simulink model "c221007_FCEV_CDCS"  (R2022b)
settings: Solver=ode4  StartTime=1  StopTime=size(Driving_cycle_v_kmph,1)  FixedStep=Auto  RelTol=1e-3  EnableMultiTasking=on
values from neighbouring files (symbols this model uses):
  Bat_eff_chg_average = 0.969    [FCEV_original_data.mat]
  Bat_eff_dis_average = 0.9632    [FCEV_original_data.mat]
  Bat_end_of_life_percent = 20    [FCEV_original_data.mat]
  Bat_I_chg_max = -120    [FCEV_original_data.mat]
  Bat_I_dis_max = 200    [FCEV_original_data.mat]
  Bat_nom_Ic = 2.5    [FCEV_original_data.mat]
  Bat_nom_SOC = 0.35    [FCEV_original_data.mat]
  Bat_nom_temp_oC = 25    [FCEV_original_data.mat]
  Bat_num_pa = 9    [FCEV_original_data.mat]
  Bat_num_se = 97    [FCEV_original_data.mat]
  Bat_ori_C1_chg_F = [397.526659684 455.660832136 435.08783522 460.845064365 457.605812374 417.289828504 416.373906992 359.741413056 321.561704819 1109.14132554 1165.67733205 1135.97600211 ... (72 elements, 9x8)]    [FCEV_original_data.mat]
  Bat_ori_C1_dis_F = [187.121968588 287.083505726 346.448009002 395.529439835 387.517274826 389.973134196 432.856765051 486.92921923 512.158935268 425.990733989 614.68708868 771.472592368 ... (72 elements, 9x8)]    [FCEV_original_data.mat]
  Bat_ori_C2_chg_F = [8748.48589695 7773.35875681 9404.86567646 8934.73981058 8290.58671366 7592.78422269 7759.44623103 7396.59043829 6151.35152293 16187.7227039 11721.8480541 13157.8579836 ... (72 elements, 9x8)]    [FCEV_original_data.mat]
  Bat_ori_C2_dis_F = [2939.81325553 4590.73311898 5504.93546413 5887.5077374 6534.37836712 7765.46899768 10584.7751706 10372.0508438 9238.72693885 5207.86390693 7911.43744944 8879.62137571 ... (72 elements, 9x8)]    [FCEV_original_data.mat]
  Bat_ori_cap_max_Ah = 20.7    [Config_c221218.m]    (also in Config_c230117.m; Config_c230321.m; FCEV_original_data.mat)
  Bat_ori_dUdt4 = [-0.303773584906 -0.249056603774 -0.115094339623 -0.0396226415094 0.0396226415094 0.0641509433962 0.107547169811 0.111320754717 0.0415094339623 0.0547169811321 0.130188679245]    [FCEV_original_data.mat]
  Bat_ori_R0_chg_O = [0.0771669453735 0.0731809311402 0.0726556782939 0.0729965156794 0.0731758310684 0.0742031005051 0.0721266921026 0.0714211058078 0.0714186176143 0.0374124505155 0.0354566732504 0.0345430657188 ... (72 elements, 9x8)]    [FCEV_original_data.mat]
  Bat_ori_R0_dis_O = [0.0819458671157 0.0812429476608 0.0803749674507 0.0805513601722 0.0838629023857 0.0850797840015 0.0829875518672 0.0826388888889 0.0812514106148 0.0428124986417 0.0424658903711 0.0428572670451 ... (72 elements, 9x8)]    [FCEV_original_data.mat]
  Bat_ori_R1_chg_O = [0.114339870884 0.105392753268 0.104421193553 0.109821896183 0.114868279838 0.123333154908 0.129174812826 0.149917249373 0.174896487845 0.0420560161846 0.0390948352938 0.0370122837364 ... (72 elements, 9x8)]    [FCEV_original_data.mat]
  Bat_ori_R1_dis_O = [0.304806399643 0.213604089624 0.171463520004 0.151183840498 0.140630862434 0.128795299077 0.116857791733 0.112567113582 0.106368362501 0.0943235089866 0.0730697254134 0.0611414736086 ... (72 elements, 9x8)]    [FCEV_original_data.mat]
  Bat_ori_R2_chg_O = [0.134518959939 0.17565045702 0.161100627268 0.189032232545 0.205639040497 0.226170473035 0.223651875822 0.181765694192 0.212966950836 0.073628872144 0.0788540822416 0.0792414571734 ... (72 elements, 9x8)]    [FCEV_original_data.mat]
  Bat_ori_R2_dis_O = [0.354968099904 0.285293035102 0.286338708953 0.298763853987 0.248762838155 0.178586175471 0.129047399775 0.188406991173 0.174494800676 0.131839238891 0.123225430215 0.132069033134 ... (72 elements, 9x8)]    [FCEV_original_data.mat]
  Bat_ori_SOC2 = [0 0.001 0.002 0.003 0.004 0.005 0.006 0.007 0.008 0.009 0.01 0.011 ... (1001 elements, 1x1001)]    [FCEV_original_data.mat]
  Bat_ori_SOC4 = [-0.00598301069999 0.0920117618231 0.190864167279 0.289083557951 0.387343788287 0.485011843502 0.5850485992 0.678163031937 0.774810095565 0.876684636119 0.972739524626]    [FCEV_original_data.mat]
  Bat_ori_Uoc_chg_V = [2.4478 2.54923264342 2.6007 2.6383 2.66953057366 2.69636321708 2.7197 2.74042850391 2.75906114733 2.77619379074 2.792 2.80675907757 ... (1001 elements, 1x1001)]    [FCEV_original_data.mat]
  Bat_ori_Uoc_dis_V = [1.9998 2.03916768329 2.24724374236 2.39700902919 2.48767431602 2.5476 2.5882 2.6202 2.64771773167 2.6719 2.6933 2.71251566192 ... (1001 elements, 1x1001)]    [FCEV_original_data.mat]
  Bat_ori_Uoc_V = [2.2238 2.29420016335 2.42397187118 2.5176545146 2.57860244484 2.62198160854 2.65395 2.68031425195 2.7033894395 2.72404689537 2.74265 2.75963736975 ... (1001 elements, 1x1001)]    [FCEV_original_data.mat]
  Bat_single_capacity_nom_Ah = 2.3    [FCEV_original_data.mat]
  Bat_SOC_cs_max = 0.4    [FCEV_original_data.mat]
  Bat_SOC_cs_min = 0.2    [FCEV_original_data.mat]
  Bat_SOC_ini = 0.3    [Config_c22100601.m]    (also in Config_c22100701.m; FCEV_original_data.mat = 0.45)
  Bat_SOC_max = 0.9    [FCEV_original_data.mat]
  Bat_SOC_min = 0.3    [FCEV_original_data.mat]
  Bat_temp_amb_oC = 25    [FCEV_original_data.mat]
  Bat_temp_cool_oC = 25    [FCEV_original_data.mat]
  Bat_U_avg_V = Bat_num_se*mean(Bat_ori_Uoc_V)    [Config_c22100601.m]    (also in Config_c22100701.m)
  DCAC_eff = 0.95    [FCEV_original_data.mat]
  DCDC_ori_eff = [0.95 0.96 0.97 0.976 0.98 0.978 0.973 0.962]    [FCEV_original_data.mat]
  DCDC_ori_power_kW = [0 10 20 30 40 50 60 70]    [FCEV_original_data.mat]
  FC_fuel_mass_ini_kg = 10    [FCEV_original_data.mat]
  FC_ori_eff = [0.1 0.33 0.492 0.533 0.559 0.596 0.591 0.562 0.508]    [FCEV_original_data.mat]
  FC_ori_fuel_rate_gps = [0 0.0505050505051 0.0846883468835 0.117260787992 0.149075730471 0.279642058166 0.423011844332 0.593119810202 0.820209973753]    [FCEV_original_data.mat]
  FC_ori_power_kW = [0 2 5 7.5 10 20 30 40 50]    [FCEV_original_data.mat]
  FC_power_max_kW = 50    [FCEV_original_data.mat]
  FC_power_min_kW = 0    [FCEV_original_data.mat]
  MC_eff_brk_average = 0.810578512397    [FCEV_original_data.mat]
  MC_eff_dri_average = 0.810578512397    [FCEV_original_data.mat]
  MC_inertia = 0.06    [FCEV_original_data.mat]
  MC_ori_eff = [0.7 0.78 0.85 0.86 0.81 0.82 0.79 0.78 0.78 0.78 0.78 0.7 ... (231 elements, 11x21)]    [FCEV_original_data.mat]
  MC_ori_power_brk_req_kW = [0 -28.3912930389 -56.7825860779 -85.1738791168 -113.565172156 -141.956465195 -170.347758234 -198.739051273 -227.130344311 -255.52163735 -283.912930389 0 ... (121 elements, 11x11)]    [FCEV_original_data.mat]
  MC_ori_power_dri_req_kW = [0 0 0 0 0 0 0 0 0 0 0 0 ... (121 elements, 11x11)]    [FCEV_original_data.mat]
  MC_ori_spd_rpm = [0 1000 2000 3000 4000 5000 6000 7000 8000 9000 10000]    [FCEV_original_data.mat]
  MC_ori_trq_brk_max_Nm = [-271.1368 -271.1368 -271.1368 -237.5159 -178.1369 -142.4824 -118.7579 -101.8119 -89.0685 -79.172 -71.1734]    [FCEV_original_data.mat]
  MC_ori_trq_brk_Nm = [-271.136848522 -244.02316367 -216.909478817 -189.795793965 -162.682109113 -135.568424261 -108.454739409 -81.3410545565 -54.2273697044 -27.1136848522 0]    [FCEV_original_data.mat]
  MC_ori_trq_dri_max_Nm = [271.1368 271.1368 271.1368 237.5159 178.1369 142.4824 118.7579 101.8119 89.0685 79.172 71.1734]    [FCEV_original_data.mat]
  MC_ori_trq_dri_Nm = [0 27.1136848522 54.2273697044 81.3410545565 108.454739409 135.568424261 162.682109113 189.795793965 216.909478817 244.02316367 271.136848522]    [FCEV_original_data.mat]
  MC_ori_trq_Nm = [-271.136848522 -244.02316367 -216.909478817 -189.795793965 -162.682109113 -135.568424261 -108.454739409 -81.3410545565 -54.2273697044 -27.1136848522 0 27.1136848522 ... (21 elements, 1x21)]    [FCEV_original_data.mat]
  MC_power_max_kW = 75    [FCEV_original_data.mat]
  MC_spd_max_rpm = 10000    [FCEV_original_data.mat]
  MC_spd_min_rpm = 0    [FCEV_original_data.mat]
  MC_spd_scale = 1    [FCEV_original_data.mat]
  MC_trq_scale = 1    [FCEV_original_data.mat]
  MC_U_min_V = 120    [FCEV_original_data.mat]
  Road_u = 0.75    [FCEV_original_data.mat]
  S_r = floor(max(Sr_SOC_process(:,1))):-1:0    [Config_c22100601.m]    (also in Config_c22100701.m)
  Time_sample = 60    [Driving_cycle_recognition_data.mat]
  Trip_distance_total_km = sum(Driving_cycle_v_kmph(:,2)/3.6)/1000    [Config_c22100601.m]    (also in Config_c22100701.m)
  usd2rmb = 7.116    [Config_c22100601.m]    (also in Config_c22100701.m; Config_c221106.m = 6; Config_c221112.m = 6; Config_c221127.m = 6)
  Veh_air_density_kgpm2 = 1.2    [FCEV_original_data.mat]
  Veh_brk_front = [1 0.6 0.608 0.61 0.618 0.624 0.636 0.645 0.655]    [FCEV_original_data.mat]
  Veh_brk_z = [0.1 0.2 0.3 0.4 0.5 0.6 0.7 0.8 0.9]    [FCEV_original_data.mat]
  Veh_brk_z_max = 0.7    [FCEV_original_data.mat]
  Veh_brk_z_min = 0.1    [FCEV_original_data.mat]
  Veh_coeff_drag = 0.312    [FCEV_original_data.mat]
  Veh_coeff_roll = 0.00863    [FCEV_original_data.mat]
  Veh_final_drive_inertia = 0.1105    [FCEV_original_data.mat]
  Veh_final_drive_ratio = 3.47    [FCEV_original_data.mat]
  Veh_frontal_area_m2 = 2.06    [FCEV_original_data.mat]
  Veh_gravity_acc_ms2 = 9.81    [FCEV_original_data.mat]
  Veh_mass_cargo_kg = 113    [FCEV_original_data.mat]
  Veh_mass_curb_kg = 1157    [FCEV_original_data.mat]
  Veh_mech_eff = 0.9    [FCEV_original_data.mat]
  Veh_rotary_mass_conversion_factor = 1.05    [FCEV_original_data.mat]
  Veh_size_cg_height_m = 0.53    [FCEV_original_data.mat]
  Veh_wheel_inertia = 3.1039    [FCEV_original_data.mat]
  Veh_wheel_radius_m = 0.313    [FCEV_original_data.mat]
  Veh_wt_frac_front = 0.5    [FCEV_original_data.mat]
undefined symbols (not defined in the file or in its folder): alpha, Bat_ori_temp, Sr_e
libraries: neural x10
(part 3 of 5)

== system c221007_FCEV_CDCS/燃料电池模型/FcDegCountingSubSys/Subsystem ==
  Enable : EnablePort
  Add : Sum
  Constant : Constant
  Memory : Memory
  u : Outport
  wires:
  Constant/1 -> Add/1
  Add/1 -> Memory/1
  Memory/1 -> Add/2, u/1

== system c221007_FCEV_CDCS/燃料电池模型/FcDegCountingSubSys/Subsystem1 ==
  Enable : EnablePort
  Add : Sum
  Constant : Constant
  Memory : Memory
  u : Outport
  wires:
  Memory/1 -> u/1, Add/2
  Add/1 -> Memory/1
  Constant/1 -> Add/1

== system c221007_FCEV_CDCS/电池模型/Capacity Degradation Model (Cell)/计算实际寿命 ==
  note: 参考文献：A control-oriented cycle-life model for hybrid electric vehicle lithiumion batteries
  note: Beta
  note: Alpha
  温度 : Inport
  倍率 : Inport  Port=2
  SOC : Inport  Port=3
  -31700+163.3*Ic : Sum  InputSameDT=on  SaturateOnIntegerOverflow=on  OutDataTypeStr=Inherit: Same as first input
  Alpha*SOC+Beta1 : Sum  InputSameDT=on  SaturateOnIntegerOverflow=on  OutDataTypeStr=Inherit: Same as first input
  Alpha3 : Constant  Value=2896.6
  Alpha4 : Constant  Value=2649.5
  Beta3 : Constant  Value=7411.2
  Beta4 : Constant  Value=6022.2
  Constant : Constant  Value=-31500
  Constant1 : Constant  Value=152.5
  Constant2 : Constant  Value=273.15
  Fcn2 : Fcn  Expr=u^(1/0.57)
  Math Function : Math  Operator=reciprocal  SignedPower=on
  Math Function1 : Math  Operator=reciprocal  SignedPower=on
  Math Function2 : Math  SignedPower=on
  R : Constant  Value=8.314
  R*T : Product  InputSameDT=on  RndMeth=Zero  SaturateOnIntegerOverflow=on  OutDataTypeStr=Inherit: Same as first input
  Switch3 : Switch  Criteria=u2 > Threshold  Threshold=0.45
  Switch4 : Switch  Criteria=u2 > Threshold  Threshold=0.45
  severity factor function : Product  InputSameDT=on  RndMeth=Zero  SaturateOnIntegerOverflow=on  OutDataTypeStr=Inherit: Same as first input
  x : Product  InputSameDT=on  RndMeth=Zero  SaturateOnIntegerOverflow=on  OutDataTypeStr=Inherit: Same as first input
  x1 : Product  InputSameDT=on  RndMeth=Zero  SaturateOnIntegerOverflow=on  OutDataTypeStr=Inherit: Same as first input
  x2 : Product  InputSameDT=on  RndMeth=Zero  SaturateOnIntegerOverflow=on  OutDataTypeStr=Inherit: Same as first input
  ×1 : Product  InputSameDT=on  RndMeth=Zero  SaturateOnIntegerOverflow=on  OutDataTypeStr=Inherit: Same as first input
  ℃->开氏温度(绝对温度) : Sum  InputSameDT=on  SaturateOnIntegerOverflow=on  OutDataTypeStr=Inherit: Same as first input
  电池标准状态寿命 : ToWorkspace  VariableName=Bat_life_nom  SampleTime=-1
  电池终止寿命(%) : Constant  Value=Bat_end_of_life_percent
  Bat_life_nom : Outport
  wires:
  R/1 -> R*T/1
  ℃->开氏温度(绝对温度)/1 -> R*T/2
  Constant/1 -> -31700+163.3*Ic/1
  x/1 -> -31700+163.3*Ic/2
  Constant1/1 -> x/1
  -31700+163.3*Ic/1 -> x1/1
  R*T/1 -> Math Function/1
  Math Function/1 -> x1/2
  x1/1 -> Math Function2/1
  温度/1 -> ℃->开氏温度(绝对温度)/1
  Constant2/1 -> ℃->开氏温度(绝对温度)/2
  倍率/1 -> x/2
  Math Function2/1 -> severity factor function/1
  Alpha*SOC+Beta1/1 -> severity factor function/2
  severity factor function/1 -> Math Function1/1
  电池终止寿命(%)/1 -> x2/1
  Math Function1/1 -> x2/2
  x2/1 -> Fcn2/1
  Fcn2/1 -> Bat_life_nom/1, 电池标准状态寿命/1
  SOC/1 -> Switch4/2, ×1/1, Switch3/2
  Alpha4/1 -> Switch3/1
  Alpha3/1 -> Switch3/3
  Beta4/1 -> Switch4/1
  Beta3/1 -> Switch4/3
  Switch3/1 -> ×1/2
  Switch4/1 -> Alpha*SOC+Beta1/2
  ×1/1 -> Alpha*SOC+Beta1/1

== system c221007_FCEV_CDCS/电池模型/Capacity Degradation Model (Cell)/计算电池寿命(标准条件下) ==
  note: 参考文献：A control-oriented cycle-life model for hybrid electric vehicle lithiumion batteries
  note: Beta
  note: Alpha
  标准温度 : Inport
  标准倍率 : Inport  Port=2
  标准SOC : Inport  Port=3
  -31500+152.5*Ic : Sum  InputSameDT=on  SaturateOnIntegerOverflow=on  OutDataTypeStr=Inherit: Same as first input
  Alpha*SOC+Beta : Sum  InputSameDT=on  SaturateOnIntegerOverflow=on  OutDataTypeStr=Inherit: Same as first input
  Alpha3 : Constant  Value=2896.6
  Alpha4 : Constant  Value=2649.5
  Beta3 : Constant  Value=7411.2
  Beta4 : Constant  Value=6022.2
  Constant : Constant  Value=-31500
  Constant1 : Constant  Value=152.5
  Constant2 : Constant  Value=273.15
  Fcn2 : Fcn  Expr=u^(1/0.57)
  Math Function : Math  Operator=reciprocal  SignedPower=on
  Math Function1 : Math  Operator=reciprocal  SignedPower=on
  Math Function2 : Math  SignedPower=on
  R : Constant  Value=8.314
  R*T : Product  InputSameDT=on  RndMeth=Zero  SaturateOnIntegerOverflow=on  OutDataTypeStr=Inherit: Same as first input
  Switch3 : Switch  Criteria=u2 > Threshold  Threshold=0.45
  Switch4 : Switch  Criteria=u2 > Threshold  Threshold=0.45
  severity factor function : Product  InputSameDT=on  RndMeth=Zero  SaturateOnIntegerOverflow=on  OutDataTypeStr=Inherit: Same as first input
  x : Product  InputSameDT=on  RndMeth=Zero  SaturateOnIntegerOverflow=on  OutDataTypeStr=Inherit: Same as first input
  x1 : Product  InputSameDT=on  RndMeth=Zero  SaturateOnIntegerOverflow=on  OutDataTypeStr=Inherit: Same as first input
  x2 : Product  InputSameDT=on  RndMeth=Zero  SaturateOnIntegerOverflow=on  OutDataTypeStr=Inherit: Same as first input
  ×1 : Product  InputSameDT=on  RndMeth=Zero  SaturateOnIntegerOverflow=on  OutDataTypeStr=Inherit: Same as first input
  ℃->开氏温度(绝对温度) : Sum  InputSameDT=on  SaturateOnIntegerOverflow=on  OutDataTypeStr=Inherit: Same as first input
  电池实际状态寿命 : ToWorkspace  VariableName=Bat_life_act  SampleTime=-1
  电池终止寿命(%) : Constant  Value=Bat_end_of_life_percent
  Bat_life_act : Outport
  wires:
  R/1 -> R*T/1
  ℃->开氏温度(绝对温度)/1 -> R*T/2
  Constant/1 -> -31500+152.5*Ic/1
  x/1 -> -31500+152.5*Ic/2
  Constant1/1 -> x/1
  -31500+152.5*Ic/1 -> x1/1
  R*T/1 -> Math Function/1
  Math Function/1 -> x1/2
  x1/1 -> Math Function2/1
  标准温度/1 -> ℃->开氏温度(绝对温度)/1
  Constant2/1 -> ℃->开氏温度(绝对温度)/2
  标准倍率/1 -> x/2
  Math Function2/1 -> severity factor function/1
  Alpha*SOC+Beta/1 -> severity factor function/2
  severity factor function/1 -> Math Function1/1
  电池终止寿命(%)/1 -> x2/1
  Math Function1/1 -> x2/2
  x2/1 -> Fcn2/1
  Fcn2/1 -> Bat_life_act/1, 电池实际状态寿命/1
  标准SOC/1 -> Switch4/2, ×1/1, Switch3/2
  Alpha4/1 -> Switch3/1
  Alpha3/1 -> Switch3/3
  Beta4/1 -> Switch4/1
  Beta3/1 -> Switch4/3
  Switch3/1 -> ×1/2
  Switch4/1 -> Alpha*SOC+Beta/2
  ×1/1 -> Alpha*SOC+Beta/1

== system c221007_FCEV_CDCS/电池模型/Electrical Model/Current calculation ==
  note: #:电池单体水平
  note: R0chg
  note: R0dis
  Voc : Inport
  Rint : Inport  Port=2
  limited output power (W) : Inport  Port=3
  Constant : Constant  Value=Bat_I_chg_max
  Constant1 : Constant  Value=Bat_I_dis_max
  Constant2 : Constant  Value=0
  Demux : Demux  Outputs=2
  Ibty=(Voc-(Voc^2-4RPbty)^.5) ----------------------------- (2*R) : Fcn  Expr=(u[2]-(u[2]^2-4*u[1]*u[3])^.5)/(2*u[3])
  Ibty=(Voc-(Voc^2-4RPbty)^.5) ----------------------------- (2*R)1 : Fcn  Expr=(u[2]-(u[2]^2-4*u[1]*u[3])^.5)/(2*u[3])
  MinMax : MinMax  Inputs=2
  MinMax1 : MinMax  Function=max  Inputs=2
  Mux : Mux  Inputs=2
  Mux1 : Mux  Inputs=3
  Mux2 : Mux  Inputs=3
  Pbat->Pcell : Gain  Gain=1/(Bat_num_pa*Bat_num_se)  SaturateOnIntegerOverflow=on  OutDataTypeStr=Inherit: Same as input  ParamDataTypeStr=Inherit: Same as input
  Scope : Scope
  Scope1 : Scope
  Switch : Switch  Criteria=u2 > Threshold
  Switch1 : Switch  Criteria=u2 > Threshold  SaturateOnIntegerOverflow=off  InputSameDT=off
  Switch2 : Switch  Criteria=u2 > Threshold
  I_dis (A) I_chg (A) Cell : Outport  InitialOutput=0
  I (A) Cell : Outport  Port=2  InitialOutput=0
  wires:
  Rint/1 -> Demux/1
  limited output power (W)/1 -> Pbat->Pcell/1
  Pbat->Pcell/1 -> Switch/1, Switch/2, Switch2/3, Switch2/2, Switch1/2
  Mux1/1 -> Ibty=(Voc-(Voc^2-4RPbty)^.5) ----------------------------- (2*R)/1
  Demux/1 -> Mux1/3
  Voc/1 -> Mux1/2, Mux2/2
  Demux/2 -> Mux2/3
  Mux2/1 -> Ibty=(Voc-(Voc^2-4RPbty)^.5) ----------------------------- (2*R)1/1
  Ibty=(Voc-(Voc^2-4RPbty)^.5) ----------------------------- (2*R)/1 -> MinMax/2
  Constant1/1 -> MinMax/1
  Ibty=(Voc-(Voc^2-4RPbty)^.5) ----------------------------- (2*R)1/1 -> MinMax1/1
  Constant/1 -> MinMax1/2
  MinMax/1 -> Switch1/1, Mux/1
  MinMax1/1 -> Mux/2, Switch1/3
  Mux/1 -> Scope/1, I_dis (A) I_chg (A) Cell/1
  Switch1/1 -> Scope1/1, I (A) Cell/1
  Switch/1 -> Mux1/1
  Switch2/1 -> Mux2/1
  Constant2/1 -> Switch/3, Switch2/1

== system c221007_FCEV_CDCS/电池模型/Electrical Model/Entropic Heat ==
  note: 用于计算可逆热
  T : Inport
  SOC : Inport  Port=2
  Constant : Constant  Value=273
  Ent heat : Product  RndMeth=Zero
  Scope : Scope
  Sum2 : Sum  Inputs=|++
  dudT : Lookup  InputValues=Bat_ori_SOC4  Table=Bat_ori_dUdt4  SaturateOnIntegerOverflow=off
  mV->V : Gain  Gain=1/1000
  HG_ent : Outport
  wires:
  Sum2/1 -> Ent heat/2
  Constant/1 -> Sum2/2
  T/1 -> Sum2/1
  dudT/1 -> Ent heat/1
  Ent heat/1 -> mV->V/1
  SOC/1 -> dudT/1
  mV->V/1 -> Scope/1, HG_ent/1

== system c221007_FCEV_CDCS/电池模型/Electrical Model/Limited power (Battery pack level) ==
  SOC : Inport
  Pbty : Inport  Port=2
  " " : RelationalOperator  Operator=>  OutDataTypeStr=boolean  InputSameDT=off
  " 1" : RelationalOperator  Operator=<  OutDataTypeStr=boolean  InputSameDT=off
  " 3" : Constant  Value=0.95
  Add : Sum
  Constant : Constant  Value=eps
  Constant1 : Constant  Value=eps
  Constant{2..5} (4 alike) : Constant  Value=0
  Logical Operator : Logic  Operator=OR  AllPortsSameDT=off  OutDataTypeStr=boolean
  Logical Operator1 : Logic  AllPortsSameDT=off  OutDataTypeStr=boolean
  Memory1 : Memory  InitialCondition=Bat_SOC_ini  InheritSampleTime=on
  Relational Operator : RelationalOperator  Operator=>  OutDataTypeStr=boolean  InputSameDT=off
  Relational Operator1 : RelationalOperator  OutDataTypeStr=boolean  InputSameDT=off
  Scope : Scope
  Scope1 : Scope  NumInputPorts=2
  Scope2 : Scope  NumInputPorts=2
  Scope3 : Scope
  Switch{,1..3} (4 alike) : Switch  Criteria=u2 > Threshold  Threshold=eps  SaturateOnIntegerOverflow=off  InputSameDT=off
  "Pbty, limited W" : Outport  InitialOutput=0
  wires:
  Memory1/1 -> Relational Operator/1, Relational Operator1/1, Scope3/1
  Constant/1 -> Relational Operator/2
  Relational Operator/1 -> Logical Operator/1
  Switch3/1 -> Scope2/2, " 1"/1, Switch1/3
  Constant1/1 -> " "/2
  " "/1 -> Logical Operator/2
  Logical Operator/1 -> Switch/2
  Constant2/1 -> Switch/3
  " 3"/1 -> Relational Operator1/2
  Relational Operator1/1 -> Logical Operator1/1
  Logical Operator1/1 -> Switch1/2
  Constant3/1 -> Switch1/1
  Constant4/1 -> " 1"/2
  " 1"/1 -> Logical Operator1/2
  Switch2/1 -> Scope2/1, " "/1, Switch/1
  Add/1 -> Scope/1, "Pbty, limited W"/1
  Switch/1 -> Scope1/1, Add/1
  Switch1/1 -> Add/2, Scope1/2
  Pbty/1 -> Switch3/3, Switch3/2, Switch2/1, Switch2/2
  Constant5/1 -> Switch3/1, Switch2/3
  SOC/1 -> Memory1/1

== system c221007_FCEV_CDCS/电池模型/Electrical Model/Max power in W (Battery pack level) ==
  Constant3 : Constant  Value=Bat_I_dis_max
  Constant4 : Constant  Value=Bat_I_chg_max
  Max power in W (Battery pack level)1 : Subsystem
  Mux1 : Mux  Inputs=3
  Mux2 : Mux  Inputs=3
  Product : Product  InputSameDT=on  RndMeth=Zero  SaturateOnIntegerOverflow=on  OutDataTypeStr=Inherit: Same as first input
  Product1 : Product  InputSameDT=on  RndMeth=Zero  SaturateOnIntegerOverflow=on  OutDataTypeStr=Inherit: Same as first input
  R0,cell->R0,bat : Gain  Gain=Bat_num_se/Bat_num_pa  SaturateOnIntegerOverflow=on  OutDataTypeStr=Inherit: Same as input  ParamDataTypeStr=Inherit: Same as input
  R0,cell->R0,bat1 : Gain  Gain=Bat_num_se/Bat_num_pa  SaturateOnIntegerOverflow=on  OutDataTypeStr=Inherit: Same as input  ParamDataTypeStr=Inherit: Same as input
  fun : Fcn  Expr=u[2]-u[1]*u[3]
  fun1 : Fcn  Expr=u[2]-u[1]*u[3]
  max ess discharge pwr : Outport  InitialOutput=0
  max ess charge pwr : Outport  Port=2  InitialOutput=0
  wires:
  [Bat_R0_dis_O] -> R0,cell->R0,bat/1
  [Bat_R0_chg_O] -> R0,cell->R0,bat1/1
  Constant4/1 -> Product1/1, Mux2/1
  Constant3/1 -> Product/1, Mux1/1
  R0,cell->R0,bat/1 -> Mux1/3
  [Bat_Uoc_V] -> Mux2/2, Mux1/2
  Mux1/1 -> fun/1
  R0,cell->R0,bat1/1 -> Mux2/3
  Mux2/1 -> fun1/1
  fun/1 -> Product/2
  Product/1 -> max ess discharge pwr/1
  fun1/1 -> Product1/2
  Product1/1 -> max ess charge pwr/1

== system c221007_FCEV_CDCS/电池模型/Electrical Model/Parameter Lookup2 ==
  note: #Cell层面
  SOC : Inport
  T : Inport  Port=2
  P : Inport  Port=3
  Gain{1..5} (5 alike) : Gain
  Lookup C1 : Subsystem
  Lookup C2 : Subsystem
  Lookup R1 : Subsystem
  Lookup R2 : Subsystem
  Lookup Rs : Subsystem
  Lookup Uoc : Subsystem
  Uoc : Outport
  R1 : Outport  Port=2
  C1 : Outport  Port=3
  R2 : Outport  Port=4
  C2 : Outport  Port=5
  R0 : Outport  Port=6
  wires:
  SOC/1 -> Lookup Rs/1(SOC), Lookup R1/1(SOC), Lookup C1/1(SOC), Lookup Uoc/1(SOC), Lookup C2/1(SOC), Lookup R2/1(SOC1)
  T/1 -> Lookup Rs/2(T), Lookup R1/2(T), Lookup C1/2(T), Lookup C2/2(T), Lookup R2/2(T)
  P/1 -> Lookup R1/3(P), Lookup C1/3(P), Lookup C2/3(P), Lookup Uoc/2(P), Lookup R2/3(P)
  Gain3/1 -> C1/1
  Lookup C2/1(C2) -> Gain4/1
  Gain4/1 -> C2/1
  Gain2/1 -> R2/1
  Lookup R2/1(R2) -> Gain2/1
  Gain1/1 -> R1/1
  Lookup R1/1(R1) -> Gain1/1
  Lookup C1/1(C1) -> Gain3/1
  Lookup Uoc/1(Uoc) -> Gain5/1
  Gain5/1 -> Uoc/1
  Lookup Rs/1(R0) -> R0/1

== system c221007_FCEV_CDCS/电池模型/Electrical Model/SOC Calculation ==
  note: 充电
  note: 放电
  note: #:电池组水平
  I_dis (A) I_chg (A) : Inport
  (sec->hrs) : Gain  Gain=1/3600  SaturateOnIntegerOverflow=on  OutDataTypeStr=Inherit: Same as input  ParamDataTypeStr=Inherit: Same as input
  0 <= SOC <= 1 : Saturate  UpperLimit=1  LowerLimit=eps
  Add5 : Sum  Inputs=-+
  Add6 : Sum  Inputs=-+
  Bat SOC0 : Constant  Value=Bat_SOC_ini
  Bat chg eff : Constant  Value=Bat_eff_chg_average
  Bat dis eff : Constant  Value=Bat_eff_dis_average
  CD/CS mode judgement : Subsystem
  Demux : Demux  Outputs=2
  Divide1 : Product  Inputs=*/
  Divide3 : Product  Inputs=**
  Divide4 : Product  Inputs=*/
  Icell->Ibat : Gain  Gain=Bat_num_pa  SaturateOnIntegerOverflow=on  OutDataTypeStr=Inherit: Same as input  ParamDataTypeStr=Inherit: Same as input
  Icell->Ibat1 : Gain  Gain=Bat_num_pa  SaturateOnIntegerOverflow=on  OutDataTypeStr=Inherit: Same as input  ParamDataTypeStr=Inherit: Same as input
  Integrator1 : Integrator  InitialCondition=eps
  Integrator6 : Integrator
  Integrator7 : Integrator
  Product3 : Product  RndMeth=Zero
  Product4 : Product  RndMeth=Zero
  Q0 : Constant  Value=Bat_ori_cap_max_Ah
  Scope : Scope
  Switch : Switch  Criteria=u2 > Threshold  SaturateOnIntegerOverflow=off  InputSameDT=off
  To Workspace3 : ToWorkspace  VariableName=Energy_bat_consume_kWh  SaveFormat=Timeseries  SampleTime=-1
  Ws->kWh : Gain  Gain=-1/(1000*3600)
  Ws->kWh1 : Gain  Gain=-1/(1000*3600)
  SOC : Outport  InitialOutput=0
  wires:
  0 <= SOC <= 1/1 -> CD/CS mode judgement/1(SOC), SOC/1
  I_dis (A) I_chg (A)/1 -> Scope/1, Demux/1
  Demux/1 -> Icell->Ibat/1
  Demux/2 -> Icell->Ibat1/1
  Divide3/1 -> Switch/2, Product3/1, Switch/1
  Icell->Ibat/1 -> Divide3/1
  Bat dis eff/1 -> Divide3/2
  Bat chg eff/1 -> Divide4/2
  Icell->Ibat1/1 -> Divide4/1
  Divide4/1 -> Product4/2, Switch/3
  Add5/1 -> 0 <= SOC <= 1/1
  [Bat_Uoc_V] -> Product4/1, Product3/2
  Add6/1 -> To Workspace3/1
  Product3/1 -> Integrator6/1
  Integrator6/1 -> Ws->kWh/1
  Ws->kWh/1 -> Add6/1
  Product4/1 -> Integrator7/1
  Integrator7/1 -> Ws->kWh1/1
  Ws->kWh1/1 -> Add6/2
  Switch/1 -> (sec->hrs)/1
  (sec->hrs)/1 -> Integrator1/1
  Integrator1/1 -> Divide1/1
  Q0/1 -> Divide1/2
  Bat SOC0/1 -> Add5/2
  Divide1/1 -> Add5/1

== system c221007_FCEV_CDCS/电池模型/Electrical Model/U0 ==
  R0 : Inport
  I : Inport  Port=2
  Demux : Demux  Outputs=2
  Switch : Switch  Criteria=u2 > Threshold  SaturateOnIntegerOverflow=off  InputSameDT=off
  U0=I*R0 : Product  RndMeth=Zero
  U0 : Outport
  wires:
  I/1 -> U0=I*R0/2, Switch/2
  R0/1 -> Demux/1
  Demux/1 -> Switch/1
  Demux/2 -> Switch/3
  Switch/1 -> U0=I*R0/1
  U0=I*R0/1 -> U0/1

== system c221007_FCEV_CDCS/电池模型/Electrical Model/U1&U1 ==
  note: -V2/(C2*R2)+I/C2
  note: -V1/(C1*R1)+I/C1
  R1 : Inport
  C1 : Inport  Port=2
  R2 : Inport  Port=3
  C2 : Inport  Port=4
  I : Inport  Port=5
  Ib/C1 : Product  Inputs=*/  RndMeth=Zero
  Ib/C2 : Product  Inputs=*/  RndMeth=Zero
  Memory : Memory  InitialCondition=eps  InheritSampleTime=on
  Memory1 : Memory  InitialCondition=eps  InheritSampleTime=on
  R1*C1 : Product  Inputs=**  RndMeth=Zero
  R2*C2 : Product  Inputs=**  RndMeth=Zero
  Scope : Scope  NumInputPorts=2
  Scope1 : Scope
  Sum1 : Sum
  Sum2 : Sum  Inputs=|-+
  Sum3 : Sum  Inputs=+-|
  Sum4 : Sum
  U1/(R1*C1) : Product  Inputs=*/  RndMeth=Zero
  U2/(R2*C2) : Product  Inputs=*/  RndMeth=Zero
  U1 : Outport
  U2 : Outport  Port=2
  wires:
  C1/1 -> R1*C1/1, Ib/C1/2
  I/1 -> Scope1/1, Ib/C2/1, Ib/C1/1
  R1/1 -> R1*C1/2
  R1*C1/1 -> U1/(R1*C1)/2
  U1/(R1*C1)/1 -> Sum3/2
  Ib/C1/1 -> Sum3/1
  R2/1 -> R2*C2/1
  C2/1 -> Ib/C2/2, R2*C2/2
  R2*C2/1 -> U2/(R2*C2)/2
  Ib/C2/1 -> Sum2/2
  U2/(R2*C2)/1 -> Sum2/1
  Memory/1 -> U1/(R1*C1)/1, Sum1/2
  Memory1/1 -> Sum4/1, U2/(R2*C2)/1
  Sum3/1 -> Sum1/1
  Sum1/1 -> Scope/1, Memory/1, U1/1
  Sum2/1 -> Sum4/2
  Sum4/1 -> Scope/2, Memory1/1, U2/1

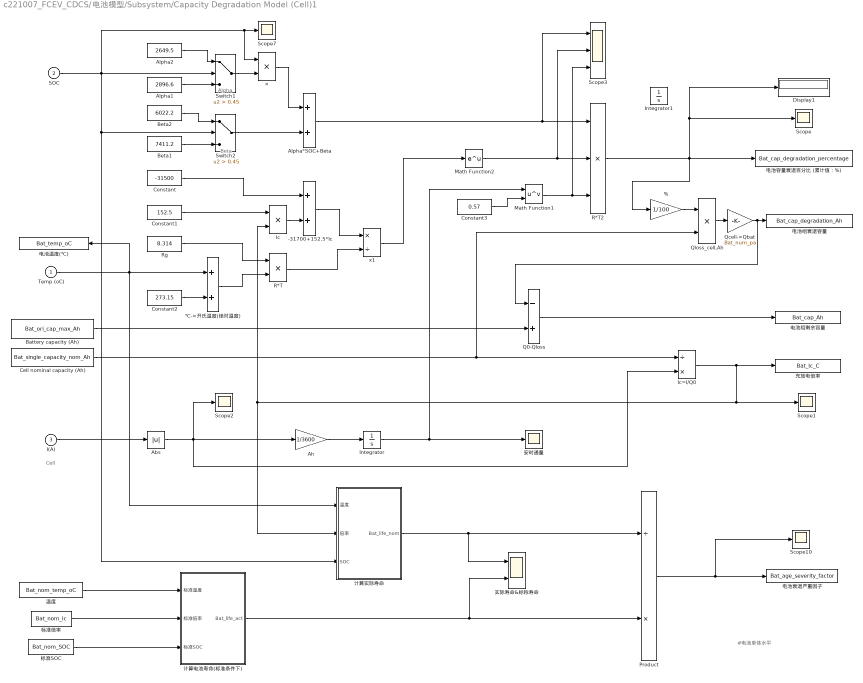
== system c221007_FCEV_CDCS/电池模型/Subsystem/Capacity Degradation Model (Cell)1 ==
  note: Cell
  note: #电池单体水平
  note: Beta
  note: Alpha
  Temp (oC) : Inport
  SOC : Inport  Port=2
  I(A) : Inport  Port=3
  % : Gain  Gain=1/100
  -31700+152.5*Ic : Sum  InputSameDT=on  SaturateOnIntegerOverflow=on  OutDataTypeStr=Inherit: Same as first input
  Abs : Abs  SaturateOnIntegerOverflow=off
  Ah : Gain  Gain=1/3600
  Alpha*SOC+Beta : Sum  InputSameDT=on  SaturateOnIntegerOverflow=on  OutDataTypeStr=Inherit: Same as first input
  Alpha1 : Constant  Value=2896.6
  Alpha2 : Constant  Value=2649.5
  Battery capacity (Ah) : Constant  Value=Bat_ori_cap_max_Ah
  Beta1 : Constant  Value=7411.2
  Beta2 : Constant  Value=6022.2
  Cell nominal capacity (Ah) : Constant  Value=Bat_single_capacity_nom_Ah
  Constant : Constant  Value=-31500
  Constant1 : Constant  Value=152.5
  Constant2 : Constant  Value=273.15
  Constant3 : Constant  Value=0.57
  Display1 : Display
  Ic : Product  InputSameDT=on  RndMeth=Zero  SaturateOnIntegerOverflow=on  OutDataTypeStr=Inherit: Same as first input
  Ic=I/Q0 : Product  Inputs=/*  InputSameDT=on  RndMeth=Zero  SaturateOnIntegerOverflow=on  OutDataTypeStr=Inherit: Same as first input
  Integrator : Integrator  InitialCondition=eps
  Integrator1 : Integrator
  Math Function1 : Math  Operator=pow  SignedPower=on
  Math Function2 : Math  SignedPower=on
  Product : Product  Inputs=/*
  Q0-Qloss : Sum  Inputs=-+  InputSameDT=on  SaturateOnIntegerOverflow=on  OutDataTypeStr=Inherit: Same as first input
  Qcell->Qbat : Gain  Gain=Bat_num_pa  SaturateOnIntegerOverflow=on  OutDataTypeStr=Inherit: Same as input  ParamDataTypeStr=Inherit: Same as input
  Qloss_cell,Ah : Product  InputSameDT=on  RndMeth=Zero  SaturateOnIntegerOverflow=on  OutDataTypeStr=Inherit: Same as first input
  R*T : Product  InputSameDT=on  RndMeth=Zero  SaturateOnIntegerOverflow=on  OutDataTypeStr=Inherit: Same as first input
  R*T2 : Product  Inputs=3  InputSameDT=on  RndMeth=Zero  SaturateOnIntegerOverflow=on  OutDataTypeStr=Inherit: Same as first input
  Rg : Constant  Value=8.314
  Scope{,1..2,7,10} (5 alike) : Scope
  Scope3 : Scope  NumInputPorts=3
  Switch1 : Switch  Criteria=u2 > Threshold  Threshold=0.45
  Switch2 : Switch  Criteria=u2 > Threshold  Threshold=0.45
  x1 : Product  Inputs=*/  InputSameDT=on  RndMeth=Zero  SaturateOnIntegerOverflow=on  OutDataTypeStr=Inherit: Same as first input
  × : Product  InputSameDT=on  RndMeth=Zero  SaturateOnIntegerOverflow=on  OutDataTypeStr=Inherit: Same as first input
  ℃->开氏温度(绝对温度) : Sum  InputSameDT=on  SaturateOnIntegerOverflow=on  OutDataTypeStr=Inherit: Same as first input
  充放电倍率 : ToWorkspace  VariableName=Bat_Ic_C  SampleTime=-1
  安时通量 : Scope
  实际寿命&标称寿命 : Scope  NumInputPorts=2
  标准SOC : Constant  Value=Bat_nom_SOC
  标准倍率 : Constant  Value=Bat_nom_Ic
  温度 : Constant  Value=Bat_nom_temp_oC  VectorParams1D=off
  电池容量衰退百分比 (累计值：%) : ToWorkspace  VariableName=Bat_cap_degradation_percentage  SampleTime=-1
  电池温度(℃) : ToWorkspace  VariableName=Bat_temp_oC  SampleTime=-1
  电池组剩余容量 : ToWorkspace  VariableName=Bat_cap_Ah  SampleTime=-1
  电池组衰退容量 : ToWorkspace  VariableName=Bat_cap_degradation_Ah  SampleTime=-1
  电池衰退严重因子 : ToWorkspace  VariableName=Bat_age_severity_factor  SampleTime=-1
  计算实际寿命 : Subsystem
  计算电池寿命(标准条件下) : Subsystem
  wires:
  SOC/1 -> Switch1/2, Scope7/1, ×/1, Switch2/2, 计算实际寿命/3(SOC)
  Alpha2/1 -> Switch1/1
  Alpha1/1 -> Switch1/3
  Beta2/1 -> Switch2/1
  Beta1/1 -> Switch2/3
  Switch1/1 -> ×/2
  Switch2/1 -> Alpha*SOC+Beta/2
  ×/1 -> Alpha*SOC+Beta/1
  Rg/1 -> R*T/1
  ℃->开氏温度(绝对温度)/1 -> R*T/2
  Ic=I/Q0/1 -> Scope1/1, Ic/2, 计算实际寿命/2(倍率), 充放电倍率/1
  Alpha*SOC+Beta/1 -> R*T2/1, Scope3/1
  Constant/1 -> -31700+152.5*Ic/1
  Ic/1 -> -31700+152.5*Ic/2
  Constant1/1 -> Ic/1
  -31700+152.5*Ic/1 -> x1/1
  R*T/1 -> x1/2
  Math Function2/1 -> R*T2/2, Scope3/2
  x1/1 -> Math Function2/1
  Math Function1/1 -> R*T2/3, Scope3/3
  R*T2/1 -> Scope/1, Display1/1, 电池容量衰退百分比 (累计值：%)/1, %/1
  Abs/1 -> Ic=I/Q0/2, Ah/1, Scope2/1
  Integrator/1 -> Math Function1/1, 安时通量/1
  Temp (oC)/1 -> 计算实际寿命/1(温度), 电池温度(℃)/1, ℃->开氏温度(绝对温度)/1
  Constant2/1 -> ℃->开氏温度(绝对温度)/2
  %/1 -> Qloss_cell,Ah/1
  温度/1 -> 计算电池寿命(标准条件下)/1(标准温度)
  标准倍率/1 -> 计算电池寿命(标准条件下)/2(标准倍率)
  标准SOC/1 -> 计算电池寿命(标准条件下)/3(标准SOC)
  Product/1 -> 电池衰退严重因子/1, Scope10/1
  计算实际寿命/1(Bat_life_nom) -> 实际寿命&标称寿命/1, Product/1
  计算电池寿命(标准条件下)/1(Bat_life_act) -> Product/2, 实际寿命&标称寿命/2
  I(A)/1 -> Abs/1
  Cell nominal capacity (Ah)/1 -> Qloss_cell,Ah/2, Ic=I/Q0/1
  Qcell->Qbat/1 -> Q0-Qloss/1, 电池组衰退容量/1
  Qloss_cell,Ah/1 -> Qcell->Qbat/1
  Battery capacity (Ah)/1 -> Q0-Qloss/2
  Q0-Qloss/1 -> 电池组剩余容量/1
  Ah/1 -> Integrator/1
  Constant3/1 -> Math Function1/2

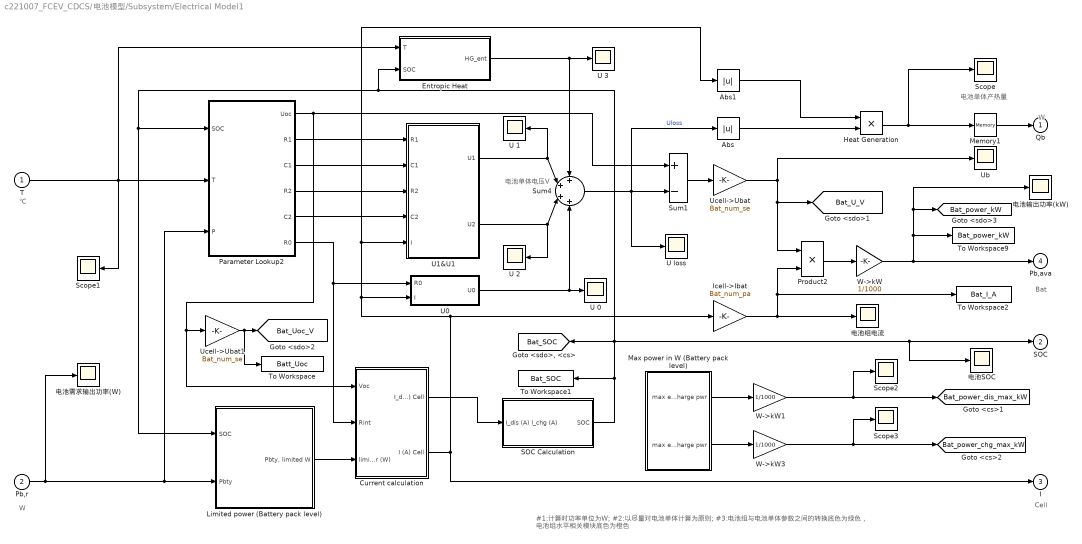
== system c221007_FCEV_CDCS/电池模型/Subsystem/Electrical Model1 ==
  note: Bat
  note: Cell
  note: W
  note: ℃
  note: #1:计算时功率单位为W;
      | #2:以尽量对电池单体计算为原则;
      | #3:电池组与电池单体参数之间的转换底色为绿色， 电池组水平相关模块底色为橙色
  note: W
  note: 电池单体产热量
  note: 电池单体电压V
  T : Inport
  Pb,r : Inport  Port=2
  Abs : Abs  SaturateOnIntegerOverflow=off
  Abs1 : Abs  SaturateOnIntegerOverflow=off
  Current calculation : Subsystem
  Entropic Heat : Subsystem
  Heat Generation : Product  RndMeth=Zero
  Icell->Ibat : Gain  Gain=Bat_num_pa  SaturateOnIntegerOverflow=on  OutDataTypeStr=Inherit: Same as input  ParamDataTypeStr=Inherit: Same as input
  Limited power (Battery pack level) : Subsystem
  Max power in W (Battery pack level) : Subsystem
  Memory1 : Memory  InheritSampleTime=on
  Parameter Lookup2 : Subsystem
  Product2 : Product  RndMeth=Zero
  SOC Calculation : Subsystem
  Scope{,1..3} (4 alike) : Scope
  Sum1 : Sum  Inputs=+-
  Sum4 : Sum  Inputs=++++
  To Workspace : ToWorkspace  VariableName=Batt_Uoc  SaveFormat=Timeseries  SampleTime=-1
  To Workspace1 : ToWorkspace  VariableName=Bat_SOC  SampleTime=-1
  To Workspace2 : ToWorkspace  VariableName=Bat_I_A  SampleTime=-1
  To Workspace9 : ToWorkspace  VariableName=Bat_power_kW  SampleTime=-1
  U {0..3} (4 alike) : Scope
  U loss : Scope
  U0 : Subsystem
  U1&U1 : Subsystem
  Ub : Scope
  Ucell->Ubat : Gain  Gain=Bat_num_se  SaturateOnIntegerOverflow=on  OutDataTypeStr=Inherit: Same as input  ParamDataTypeStr=Inherit: Same as input
  Ucell->Ubat1 : Gain  Gain=Bat_num_se  SaturateOnIntegerOverflow=on  OutDataTypeStr=Inherit: Same as input  ParamDataTypeStr=Inherit: Same as input
  W->kW : Gain  Gain=1/1000  SaturateOnIntegerOverflow=on  OutDataTypeStr=Inherit: Same as input  ParamDataTypeStr=Inherit: Same as input
  W->kW1 : Gain  Gain=1/1000  SaturateOnIntegerOverflow=on  OutDataTypeStr=Inherit: Same as input  ParamDataTypeStr=Inherit: Same as input
  W->kW3 : Gain  Gain=1/1000  SaturateOnIntegerOverflow=on  OutDataTypeStr=Inherit: Same as input  ParamDataTypeStr=Inherit: Same as input
  电池SOC : Scope
  电池组电流 : Scope
  电池输出功率(kW) : Scope
  电池需求输出功率(W) : Scope
  Qb : Outport  InitialOutput=0
  SOC : Outport  Port=2  InitialOutput=0
  I : Outport  Port=3  InitialOutput=0
  Pb,ava : Outport  Port=4  InitialOutput=0
  tag scope: Bat_SOC=global, Bat_U_V=global, Bat_Uoc_V=global, Bat_power_chg_max_kW=global, Bat_power_dis_max_kW=global, Bat_power_kW=global
  wires:
  Parameter Lookup2/2(R1) -> U1&U1/1(R1)
  Parameter Lookup2/3(C1) -> U1&U1/2(C1)
  Parameter Lookup2/4(R2) -> U1&U1/3(R2)
  Parameter Lookup2/5(C2) -> U1&U1/4(C2)
  Parameter Lookup2/6(R0) -> U0/1(R0), Current calculation/2(Rint)
  U1&U1/1(U1) -> Sum4/2, U 1/1
  U1&U1/2(U2) -> U 2/1, Sum4/3
  Ucell->Ubat/1 -> Product2/1, [Bat_U_V], Ub/1
  Entropic Heat/1(HG_ent) -> U 3/1, Sum4/1
  Product2/1 -> W->kW/1
  W->kW/1 -> 电池输出功率(kW)/1, [Bat_power_kW], To Workspace9/1, Pb,ava/1
  Memory1/1 -> Qb/1
  Heat Generation/1 -> Scope/1, Memory1/1
  Current calculation/1(I_dis (A) I_chg (A) Cell) -> SOC Calculation/1(I_dis (A) I_chg (A))
  T/1 -> Scope1/1, Entropic Heat/1(T), Parameter Lookup2/2(T)
  Pb,r/1 -> 电池需求输出功率(W)/1, Limited power (Battery pack level)/2(Pbty), Parameter Lookup2/3(P)
  Icell->Ibat/1 -> Product2/2, To Workspace2/1, 电池组电流/1
  W->kW1/1 -> Scope2/1, [Bat_power_dis_max_kW]
  W->kW3/1 -> Scope3/1, [Bat_power_chg_max_kW]
  Max power in W (Battery pack level)/1(max ess discharge pwr) -> W->kW1/1
  Max power in W (Battery pack level)/2(max ess charge pwr) -> W->kW3/1
  Parameter Lookup2/1(Uoc) -> Sum1/1, Ucell->Ubat1/1, Current calculation/1(Voc)
  Ucell->Ubat1/1 -> To Workspace/1, [Bat_Uoc_V]
  Limited power (Battery pack level)/1("Pbty, limited W") -> Current calculation/3(limited output power (W))
  SOC Calculation/1(SOC) -> 电池SOC/1, SOC/1, [Bat_SOC], Entropic Heat/2(SOC), Limited power (Battery pack level)/1(SOC), Parameter Lookup2/1(SOC), To Workspace1/1
  Current calculation/2(I (A) Cell) -> Abs1/1, U1&U1/5(I), U0/2(I), Icell->Ibat/1, I/1
  U0/1(U0) -> U 0/1, Sum4/4
  Sum4/1 -> U loss/1, Abs/1, Sum1/2  "Uloss"
  Sum1/1 -> Ucell->Ubat/1
  Abs/1 -> Heat Generation/2
  Abs1/1 -> Heat Generation/1

== system c221007_FCEV_CDCS/电池模型/Subsystem/Thermal Model1 ==
  note: 需要设置温度初始值
  note: W
  note: Tf
  note: (k)
  note: 冷却液温度 ℃
  note: ℃
  note: ℃
  Qb : Inport
  (1-1/RsCs-1/RcCs)*Ts(k-1) : Product  Inputs=**  RndMeth=Zero
  (RC*Cc-1)*Tc(k-1)/RcCc : Product  Inputs=**  RndMeth=Zero
  (RC*Cc-1)/RcCc : Product  Inputs=*/  RndMeth=Zero
  Calculation : Subsystem
  Constant : Constant  Value=273
  Constant3 : Constant
  Math Function : Math  Operator=reciprocal  SignedPower=on
  Math Function1 : Math  Operator=reciprocal  SignedPower=on
  Qb(k-1)/Cc : Product  Inputs=*/  RndMeth=Zero
  Sum10 : Sum  Inputs=+++
  Sum11 : Sum  Inputs=+--|
  Sum3 : Sum  Inputs=+++
  Sum4 : Sum  Inputs=+-|
  Sum5 : Sum  Inputs=|+-
  Sum7 : Sum  Inputs=++|
  Sum9 : Sum  Inputs=-+|
  Tc (K) : Scope
  Tc (℃) : Scope
  Tc(k-1) : Memory  InitialCondition=Bat_temp_amb_oC+273.15  InheritSampleTime=on
  Tc(k-1)/RcCs : Product  Inputs=*/  RndMeth=Zero
  Tf/RsCs : Product  Inputs=*/  RndMeth=Zero
  Tf1 : Constant  Value=Bat_temp_cool_oC
  Ts (K) : Scope
  Ts (℃) : Scope
  Ts(k-1) : Memory  InitialCondition=Bat_temp_amb_oC+273.15  InheritSampleTime=on
  Ts(k-1)/RcCc : Product  Inputs=*/  RndMeth=Zero
  Tc. : Outport
  Ts. : Outport  Port=2
  wires:
  Calculation/1(Cc) -> Qb(k-1)/Cc/2
  Calculation/2(RcCc) -> (RC*Cc-1)/RcCc/2, Ts(k-1)/RcCc/2, Sum4/1
  Constant3/1 -> Sum11/1, Sum4/2
  Sum4/1 -> (RC*Cc-1)/RcCc/1
  Qb(k-1)/Cc/1 -> Sum3/1
  Ts(k-1)/RcCc/1 -> Sum3/2
  Tf1/1 -> Sum7/2
  Calculation/3(RsCs) -> Tf/RsCs/2, Math Function/1
  Sum7/1 -> Tf/RsCs/1
  Tf/RsCs/1 -> Sum10/1
  Calculation/4(RcCs) -> Tc(k-1)/RcCs/2, Math Function1/1
  Math Function1/1 -> Sum11/2
  Math Function/1 -> Sum11/3
  (1-1/RsCs-1/RcCs)*Ts(k-1)/1 -> Sum10/2
  Sum11/1 -> (1-1/RsCs-1/RcCs)*Ts(k-1)/1
  Tc(k-1)/RcCs/1 -> Sum10/3
  Sum3/1 -> Sum5/1, Tc(k-1)/1, Tc (K)/1
  Constant/1 -> Sum9/1, Sum5/2, Sum7/1
  Sum5/1 -> Tc (℃)/1, Tc./1
  Sum10/1 -> Sum9/2, Ts(k-1)/1, Ts (K)/1
  Sum9/1 -> Ts./1, Ts (℃)/1
  Ts(k-1)/1 -> Ts(k-1)/RcCc/1, (1-1/RsCs-1/RcCs)*Ts(k-1)/2
  (RC*Cc-1)*Tc(k-1)/RcCc/1 -> Sum3/3
  (RC*Cc-1)/RcCc/1 -> (RC*Cc-1)*Tc(k-1)/RcCc/1
  Tc(k-1)/1 -> Tc(k-1)/RcCs/1, (RC*Cc-1)*Tc(k-1)/RcCc/2
  Qb/1 -> Qb(k-1)/Cc/1

== system c221007_FCEV_CDCS/电池模型/Thermal Model/Calculation ==
  Cc1 : Constant  Value=62.7
  Cs : Constant  Value=4.5
  "Rc " : Constant  Value=1.94
  Rc*Cc : Product  Inputs=**  RndMeth=Zero
  Rc*Cs : Product  Inputs=**  RndMeth=Zero
  Rs : Constant  Value=3.19
  Rs*Cs : Product  Inputs=**  RndMeth=Zero
  Cc : Outport
  RcCc : Outport  Port=2
  RsCs : Outport  Port=3
  RcCs : Outport  Port=4
  wires:
  Cc1/1 -> Cc/1, Rc*Cc/1
  "Rc "/1 -> Rc*Cc/2, Rc*Cs/1
  Rc*Cc/1 -> RcCc/1
  Cs/1 -> Rs*Cs/1, Rc*Cs/2
  Rs/1 -> Rs*Cs/2
  Rc*Cs/1 -> RcCs/1
  Rs*Cs/1 -> RsCs/1

== system c221007_FCEV_CDCS/能量管理策略 (ECMS+SQP)/Collection/    DC_type ==
  In1 : Inport
  Enable : EnablePort
  Out1 : Outport
  wires:
  In1/1 -> Out1/1

== system c221007_FCEV_CDCS/能量管理策略 (ECMS+SQP)/Collection/Bat_SOC ==
  In1 : Inport
  Enable : EnablePort
  Out1 : Outport
  wires:
  In1/1 -> Out1/1

== system c221007_FCEV_CDCS/能量管理策略 (ECMS+SQP)/Collection/Bat_SOC_max ==
  In1 : Inport
  Enable : EnablePort
  Out1 : Outport
  wires:
  In1/1 -> Out1/1

== system c221007_FCEV_CDCS/能量管理策略 (ECMS+SQP)/Collection/Bat_SOC_min ==
  In1 : Inport
  Enable : EnablePort
  Out1 : Outport
  wires:
  In1/1 -> Out1/1

== system c221007_FCEV_CDCS/能量管理策略 (ECMS+SQP)/Collection/Bat_SOC_ref ==
  In1 : Inport
  Enable : EnablePort
  Out1 : Outport
  wires:
  In1/1 -> Out1/1

== system c221007_FCEV_CDCS/能量管理策略 (ECMS+SQP)/Collection/Bat_U_avg_V ==
  In1 : Inport
  Enable : EnablePort
  Out1 : Outport
  wires:
  In1/1 -> Out1/1

== system c221007_FCEV_CDCS/能量管理策略 (ECMS+SQP)/Collection/Bat_cap_Ah ==
  In1 : Inport
  Enable : EnablePort
  Out1 : Outport
  wires:
  In1/1 -> Out1/1

== system c221007_FCEV_CDCS/能量管理策略 (ECMS+SQP)/Collection/Bat_power_max_kW ==
  In1 : Inport
  Enable : EnablePort
  Out1 : Outport
  wires:
  In1/1 -> Out1/1

== system c221007_FCEV_CDCS/能量管理策略 (ECMS+SQP)/Collection/Bat_power_min_kW ==
  In1 : Inport
  Enable : EnablePort
  Out1 : Outport
  wires:
  In1/1 -> Out1/1

== system c221007_FCEV_CDCS/能量管理策略 (ECMS+SQP)/Collection/DCAC_eff ==
  In1 : Inport
  Enable : EnablePort
  Out1 : Outport
  wires:
  In1/1 -> Out1/1

== system c221007_FCEV_CDCS/能量管理策略 (ECMS+SQP)/Collection/FC_power_max_kW ==
  In1 : Inport
  Enable : EnablePort
  Out1 : Outport
  wires:
  In1/1 -> Out1/1

== system c221007_FCEV_CDCS/能量管理策略 (ECMS+SQP)/Collection/FC_power_min_kW ==
  In1 : Inport
  Enable : EnablePort
  Out1 : Outport
  wires:
  In1/1 -> Out1/1

== system c221007_FCEV_CDCS/能量管理策略 (ECMS+SQP)/Collection/MC_power_req_kW ==
  In1 : Inport
  Enable : EnablePort
  Out1 : Outport
  wires:
  In1/1 -> Out1/1

== system c221007_FCEV_CDCS/能量管理策略 (ECMS+SQP)/Collection/X_r_km ==
  In1 : Inport
  Enable : EnablePort
  Out1 : Outport
  wires:
  In1/1 -> Out1/1

== system c221007_FCEV_CDCS/能量管理策略 (ECMS+SQP)/Collection/alpha ==
  In1 : Inport
  Enable : EnablePort
  Out1 : Outport
  wires:
  In1/1 -> Out1/1

== system c221007_FCEV_CDCS/能量管理策略 (ECMS+SQP)/FC on/Subsystem ==
  in_1 : Inport
  Constant1 : Constant  Value=n
  Integrator : Integrator
  Product : Product  Inputs=*/  InputSameDT=on  RndMeth=Zero  SaturateOnIntegerOverflow=on  OutDataTypeStr=Inherit: Same as first input
  Sum : Sum  Inputs=+-  InputSameDT=on  SaturateOnIntegerOverflow=on  OutDataTypeStr=Inherit: Same as first input
  Transport Delay : TransportDelay  DelayTime=n
  out_1 : Outport  InitialOutput=0
  wires:
  Integrator/1 -> Sum/1, Transport Delay/1
  Transport Delay/1 -> Sum/2
  Sum/1 -> Product/1
  in_1/1 -> Integrator/1
  Product/1 -> out_1/1
  Constant1/1 -> Product/2

== system c221007_FCEV_CDCS/能量管理策略 (ECMS+SQP)/FC on/dt ==
  Clock : Clock
  Memory1 : Memory  InitialCondition=-1
  Sum1 : Sum  Inputs=+-  InputSameDT=on  SaturateOnIntegerOverflow=on  OutDataTypeStr=Inherit: Same as first input
  out_1 : Outport  InitialOutput=0
  wires:
  Clock/1 -> Sum1/1, Memory1/1
  Memory1/1 -> Sum1/2
  Sum1/1 -> out_1/1

== system c221007_FCEV_CDCS/能量管理策略 (ECMS+SQP)/FC on/just shut down ==
  state : Inport
  Logical Operator : Logic
  Logical Operator1 : Logic  Operator=NOT  Inputs=1
  Memory1 : Memory  InitialCondition=1  InheritSampleTime=on
  trigger : Outport  InitialOutput=0
  wires:
  Logical Operator1/1 -> Logical Operator/1
  state/1 -> Logical Operator1/1, Memory1/1
  Memory1/1 -> Logical Operator/2
  Logical Operator/1 -> trigger/1

== system c221007_FCEV_CDCS/能量管理策略 (ECMS+SQP)/FC on/no-lag Reset Integrator ==
  in_1 : Inport
  in_2 : Inport  Port=2
  in_3 : Inport  Port=3
  Constant : Constant  Value=0
  Memory : Memory  InitialCondition=initval
  Product : Product  InputSameDT=on  RndMeth=Zero  SaturateOnIntegerOverflow=on  OutDataTypeStr=Inherit: Same as first input
  Sum : Sum  InputSameDT=on  SaturateOnIntegerOverflow=on  OutDataTypeStr=Inherit: Same as first input
  Switch : Switch  Threshold=eps
  dt : Subsystem
  in_2==0 : RelationalOperator  Operator===
  out_1 : Outport  InitialOutput=0
  wires:
  in_3/1 -> Switch/3
  in_2/1 -> in_2==0/1
  in_1/1 -> Product/2
  dt/1(out_1) -> Product/1
  Product/1 -> Sum/2
  Memory/1 -> Sum/1
  Sum/1 -> Switch/1
  Switch/1 -> out_1/1, Memory/1
  in_2==0/1 -> Switch/2
  Constant/1 -> in_2==0/2

== system c221007_FCEV_CDCS/能量管理策略 (ECMS+SQP)/SQP/Power limitation ==
  Add1 : Sum  Inputs=+-
  Add2 : Sum  Inputs=-+
  MinMax : MinMax  Function=max  Inputs=2
  Pfc_min : Constant  Value=FC_power_max_kW
  Relational Operator4 : RelationalOperator  OutDataTypeStr=boolean  InputSameDT=off
  SOC_min1 : Constant  Value=Bat_SOC_min
  Saturation1 : Saturate  UpperLimit=FC_power_max_kW  LowerLimit=FC_power_min_kW  LinearizeAsGain=off
  Switch2 : Switch  Threshold=0.1  SaturateOnIntegerOverflow=off  InputSameDT=off
  Switch3 : Switch  Threshold=0.1  SaturateOnIntegerOverflow=off  InputSameDT=off
  wires:
  Relational Operator4/1 -> Switch3/2, Switch2/2
  SOC_min1/1 -> Relational Operator4/2
  ? -> Switch2/1
  ? -> Switch3/1, Add2/2, Add1/1
  Pfc_min/1 -> Add1/2
  MinMax/1 -> Add2/1, Switch2/3
  Add1/1 -> MinMax/2
  Saturation1/1 -> Switch3/3
  Add2/1 -> Saturation1/1
  [Bat_SOC] -> Relational Operator4/1
  [Bat_power_chg_max_kW] -> MinMax/1

== system c221007_FCEV_CDCS/行驶工况相关/Custom Neural Network/Layer 1 ==
  "p{1}" : Inport  PortDimensions=3
      mask Display: e = 0.06;c1 = [120 230 180]/255;c2 = ([120 230 180]+0)/(256+128);c3 = ([120 230 180]+128)/(256+128);patch([0 1 1 0],[0 0 1 1],c1);patch([0 1 1 1-e 1-e 0+e],[0 0 1 1-e 0+e 0+e],c2);patch([0 0 1 1-e 0+e 0+e],[0 1 1 1-e 1-e 0+e],c3);plot([0 1 1 0 0],[0 0 1 1 0]);
  Delays 1 : Subsystem
      mask Display: e = 0.06;c1 = [120 150 230]/255;c2 = ([120 150 230]+0)/383;c3 = ([120 150 230]+128)/383;patch([0 1 1 0],[0 0 1 1],c1);patch([0 1 1 1-e 1-e 0+e],[0 0 1 1-e 0+e 0+e],c2);patch([0 0 1 1-e 0+e 0+e],[0 1 1 1-e 1-e 0+e],c3);plot([0 1 1 0 0],[0 0 1 1 0]);disp('0');
  "IW{1,1}" : Subsystem
      mask Display: e = 0.06;c1 = [120 150 230]/255;c2 = ([120 150 230]+0)/383;c3 = ([120 150 230]+128)/383;patch([0 1 1 0],[0 0 1 1],c1);patch([0 1 1 1-e 1-e 0+e],[0 0 1 1-e 0+e 0+e],c2);patch([0 0 1 1-e 0+e 0+e],[0 1 1 1-e 1-e 0+e],c3);plot([0 1 1 0 0],[0 0 1 1 0]);disp('W');
  compet : neural/Transfer Functions/compet  layer_size=5
  netsum : Gain  SaturateOnIntegerOverflow=on  OutDataTypeStr=Inherit: Same as input  ParamDataTypeStr=Inherit: Same as input
      mask Display: e = 0.06;c1 = [120 150 230]/255;c2 = ([120 150 230]+0)/383;c3 = ([120 150 230]+128)/383;patch([0 1 1 0],[0 0 1 1],c1);patch([0 1 1 1-e 1-e 0+e],[0 0 1 1-e 0+e 0+e],c2);patch([0 0 1 1-e 0+e 0+e],[0 1 1 1-e 1-e 0+e],c3);plot([0 1 1 0 0],[0 0 1 1 0]);disp('+');
  "a{1}" : Outport  InitialOutput=[0;0;0;0;0]
      mask Display: e = 0.06;c1 = [120 230 180]/255;c2 = ([120 230 180]+0)/(256+128);c3 = ([120 230 180]+128)/(256+128);patch([0 1 1 0],[0 0 1 1],c1);patch([0 1 1 1-e 1-e 0+e],[0 0 1 1-e 0+e 0+e],c2);patch([0 0 1 1-e 0+e 0+e],[0 1 1 1-e 1-e 0+e],c3);plot([0 1 1 0 0],[0 0 1 1 0]);
  wires:
  "p{1}"/1 -> Delays 1/1("p{1}")
  Delays 1/1("pd{1,1}") -> "IW{1,1}"/1("pd{1,1}")
  "IW{1,1}"/1("iz{1,1}") -> netsum/1
  netsum/1 -> compet/1
  compet/1 -> "a{1}"/1

== system c221007_FCEV_CDCS/行驶工况相关/Custom Neural Network/Layer 2 ==
  "a{1} " : Inport  PortDimensions=5
      mask Display: e = 0.06;c1 = [120 230 180]/255;c2 = ([120 230 180]+0)/(256+128);c3 = ([120 230 180]+128)/(256+128);patch([0 1 1 0],[0 0 1 1],c1);patch([0 1 1 1-e 1-e 0+e],[0 0 1 1-e 0+e 0+e],c2);patch([0 0 1 1-e 0+e 0+e],[0 1 1 1-e 1-e 0+e],c3);plot([0 1 1 0 0],[0 0 1 1 0]);
  Delays 1 : Subsystem
      mask Display: e = 0.06;c1 = [120 150 230]/255;c2 = ([120 150 230]+0)/383;c3 = ([120 150 230]+128)/383;patch([0 1 1 0],[0 0 1 1],c1);patch([0 1 1 1-e 1-e 0+e],[0 0 1 1-e 0+e 0+e],c2);patch([0 0 1 1-e 0+e 0+e],[0 1 1 1-e 1-e 0+e],c3);plot([0 1 1 0 0],[0 0 1 1 0]);disp('0');
  "LW{2,1}" : Subsystem
      mask Display: e = 0.06;c1 = [120 150 230]/255;c2 = ([120 150 230]+0)/383;c3 = ([120 150 230]+128)/383;patch([0 1 1 0],[0 0 1 1],c1);patch([0 1 1 1-e 1-e 0+e],[0 0 1 1-e 0+e 0+e],c2);patch([0 0 1 1-e 0+e 0+e],[0 1 1 1-e 1-e 0+e],c3);plot([0 1 1 0 0],[0 0 1 1 0]);disp('W');
  netsum : Gain  SaturateOnIntegerOverflow=on  OutDataTypeStr=Inherit: Same as input  ParamDataTypeStr=Inherit: Same as input
      mask Display: e = 0.06;c1 = [120 150 230]/255;c2 = ([120 150 230]+0)/383;c3 = ([120 150 230]+128)/383;patch([0 1 1 0],[0 0 1 1],c1);patch([0 1 1 1-e 1-e 0+e],[0 0 1 1-e 0+e 0+e],c2);patch([0 0 1 1-e 0+e 0+e],[0 1 1 1-e 1-e 0+e],c3);plot([0 1 1 0 0],[0 0 1 1 0]);disp('+');
  purelin : neural/Transfer Functions/purelin
  "a{2}" : Outport  InitialOutput=[0;0;0]
      mask Display: e = 0.06;c1 = [120 230 180]/255;c2 = ([120 230 180]+0)/(256+128);c3 = ([120 230 180]+128)/(256+128);patch([0 1 1 0],[0 0 1 1],c1);patch([0 1 1 1-e 1-e 0+e],[0 0 1 1-e 0+e 0+e],c2);patch([0 0 1 1-e 0+e 0+e],[0 1 1 1-e 1-e 0+e],c3);plot([0 1 1 0 0],[0 0 1 1 0]);
  wires:
  "a{1} "/1 -> Delays 1/1("p{2}")
  Delays 1/1("pd{2,1}") -> "LW{2,1}"/1("ad{2,1}")
  "LW{2,1}"/1("lz{2,1}") -> netsum/1
  netsum/1 -> purelin/1
  purelin/1 -> "a{2}"/1

== system c221007_FCEV_CDCS/行驶工况相关/Custom Neural Network/Process Input 1 ==
  x : Inport  PortDimensions=3
      mask Display: e = 0.06;c1 = [120 230 180]/255;c2 = ([120 230 180]+0)/(256+128);c3 = ([120 230 180]+128)/(256+128);patch([0 1 1 0],[0 0 1 1],c1);patch([0 1 1 1-e 1-e 0+e],[0 0 1 1-e 0+e 0+e],c2);patch([0 0 1 1-e 0+e 0+e],[0 1 1 1-e 1-e 0+e],c3);plot([0 1 1 0 0],[0 0 1 1 0]);
  p : Outport  PortDimensions=3
      mask Display: e = 0.06;c1 = [120 230 180]/255;c2 = ([120 230 180]+0)/(256+128);c3 = ([120 230 180]+128)/(256+128);patch([0 1 1 0],[0 0 1 1],c1);patch([0 1 1 1-e 1-e 0+e],[0 0 1 1-e 0+e 0+e],c2);patch([0 0 1 1-e 0+e 0+e],[0 1 1 1-e 1-e 0+e],c3);plot([0 1 1 0 0],[0 0 1 1 0]);
  wires:
  x/1 -> p/1

== system c221007_FCEV_CDCS/行驶工况相关/Custom Neural Network/Process Output 1 ==
  a : Inport  PortDimensions=3
      mask Display: e = 0.06;c1 = [120 230 180]/255;c2 = ([120 230 180]+0)/(256+128);c3 = ([120 230 180]+128)/(256+128);patch([0 1 1 0],[0 0 1 1],c1);patch([0 1 1 1-e 1-e 0+e],[0 0 1 1-e 0+e 0+e],c2);patch([0 0 1 1-e 0+e 0+e],[0 1 1 1-e 1-e 0+e],c3);plot([0 1 1 0 0],[0 0 1 1 0]);
  y : Outport  PortDimensions=3
      mask Display: e = 0.06;c1 = [120 230 180]/255;c2 = ([120 230 180]+0)/(256+128);c3 = ([120 230 180]+128)/(256+128);patch([0 1 1 0],[0 0 1 1],c1);patch([0 1 1 1-e 1-e 0+e],[0 0 1 1-e 0+e 0+e],c2);patch([0 0 1 1-e 0+e 0+e],[0 1 1 1-e 1-e 0+e],c3);plot([0 1 1 0 0],[0 0 1 1 0]);
  wires:
  a/1 -> y/1

== system c221007_FCEV_CDCS/车轮模型/Regenerative energy compute/compute of the brk energy ==
  motor brk force in front wheel N : Inport
  wheel linear spd m/s : Inport  Port=2
  Add : Sum
  Gain1 : Gain  Gain=-1
  Memory1 : Memory  InheritSampleTime=on
  Product : Product  RndMeth=Zero
  Scope : Scope
  Ws->kWh : Gain  Gain=1/(1000*3600)
  制动能量 : ToWorkspace  VariableName=Energy_regenerative_brk_kWh  SaveFormat=Timeseries  SampleTime=-1
  "regenerative brk energy kwh " : Outport
  wires:
  motor brk force in front wheel N/1 -> Product/1
  wheel linear spd m/s/1 -> Product/2
  Product/1 -> Gain1/1
  Ws->kWh/1 -> Scope/1, 制动能量/1, "regenerative brk energy kwh "/1
  Add/1 -> Memory1/1, Ws->kWh/1
  Memory1/1 -> Add/2
  Gain1/1 -> Add/1
